simulink model "MotorControlLib"  (R2022b)
settings: Solver=FixedStepDiscrete  StartTime=0.0  StopTime=100  FixedStep=Ts  RelTol=1e-3  EnableMultiTasking=on
values from neighbouring files (symbols this model uses):
  BrkPoints : value not decoded    [MotorControl.sldd]
  CuttOffFreq_c = 4000.0    [MotorControl.sldd]
  d_q_Voltage_Limiter_max = 5.77    [MotorControl.sldd]
  dSoll = 0.0    [MotorControl.sldd]
  EMFobsLdGain = 50000.0    [MotorControl.sldd]
  EMFobsRS = 0.34    [MotorControl.sldd]
  Ki_dAxis = 180.0    [MotorControl.sldd]
  Ki_Iab_EMFobs = 0.0    [MotorControl.sldd]
  Ki_qAxis = 175.0    [MotorControl.sldd]
  Ki_Rpm = 10.0    [MotorControl.sldd]
  Kp_dAxis = 0.146    [MotorControl.sldd]
  Kp_Iab_EMFobs = 1.0    [MotorControl.sldd]
  Kp_qAxis = 0.146    [MotorControl.sldd]
  Kp_Rpm = 0.146    [MotorControl.sldd]
  MaxBckEMFVol_sat_neg = -12.0    [MotorControl.sldd]
  MaxBckEMFVol_sat_pos = 12.0    [MotorControl.sldd]
  Minus_1 = -1.0    [MotorControl.sldd]
  pwmTableData : value not decoded    [MotorControl.sldd]
  TqToIqConst = 1.0    [MotorControl.sldd]
  Ts = 5.0E-5    [MotorControl.sldd]
  TsIntern = 5.0E-5    [MotorControl.sldd]
undefined symbols (not defined in the file or in its folder): DiscIntNeverNeededParam, NumBits1, NumBits2, Slope1, Slope2
libraries: simulink x8, slpidlib x2, simulink_extras x2
(part 1 of 2)
settings Model: DataDictionary=MotorControl.sldd  NumberOfSteps=10  Creator=unix  LastModifiedBy=unix
settings SolverCC: AlgebraicLoopSolver=TrustRegion  AutoInsertRateTranBlk=on
settings OptimizationCC: DefaultParameterBehavior=Inlined  PassReuseOutputArgsAs=Individual arguments  ZeroExternalMemoryAtStartup=off  ZeroInternalMemoryAtStartup=off  EfficientFloat2IntCast=on  OptimizationLevel=level1  OptimizationCustomize=off  EfficientTunableParamExpr=on
settings DebuggingCC: ArrayBoundsChecking=warning  SignalInfNanChecking=warning  SignalRangeChecking=warning  MultiTaskDSMMsg=warning  CheckMatrixSingularityMsg=warning  IntegerOverflowMsg=error  ParameterOverflowMsg=warning  ParameterUnderflowMsg=warning  ParameterPrecisionLossMsg=none  ParameterTunabilityLossMsg=error  UnderSpecifiedDataTypeMsg=warning  UnconnectedInputMsg=warning  UnconnectedOutputMsg=warning  UnconnectedLineMsg=warning  SFMachineParentedDataDiag=warning  IntegerSaturationMsg=error
settings ModelReferenceCC: EnableRefExpFcnMdlSchedulingChecks=on
settings SFSimCC: MATLABDynamicMemAlloc=off
settings RTWCC: Description=Embedded Coder  SystemTargetFile=ert.tlc  GenCodeOnly=on  TemplateMakefile=ert_default_tmf  GenerateReport=on  IncludeHyperlinkInReport=on  LaunchReport=on  GenerateTraceInfo=on  GenerateTraceReport=on  GenerateTraceReportSl=on  GenerateTraceReportSf=on  GenerateTraceReportEml=on  DLArmComputeVersion=19.05
settings CodeAppCC: ForceParamTrailComments=on  IgnoreCustomStorageClasses=off  OperatorAnnotations=on  SimulinkDataObjDesc=on  SFDataObjDesc=on  InsertBlockDesc=on
settings ERTTargetCC: TargetLangStandard=C99 (ISO)  CodeReplacementLibrary=GNU C99 extensions  GenerateSampleERTMain=on  ArrayLayout=Row-major  GenerateASAP2=on  InlinedParameterPlacement=NonHierarchical  ERTCustomFileTemplate=example_file_process.tlc

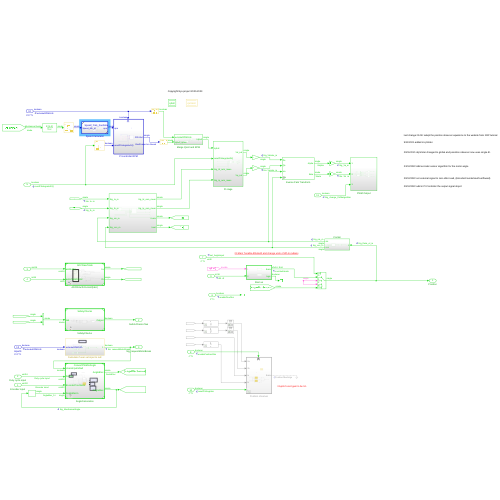
[thumbnail: Simulink's stored preview of the top-level diagram]
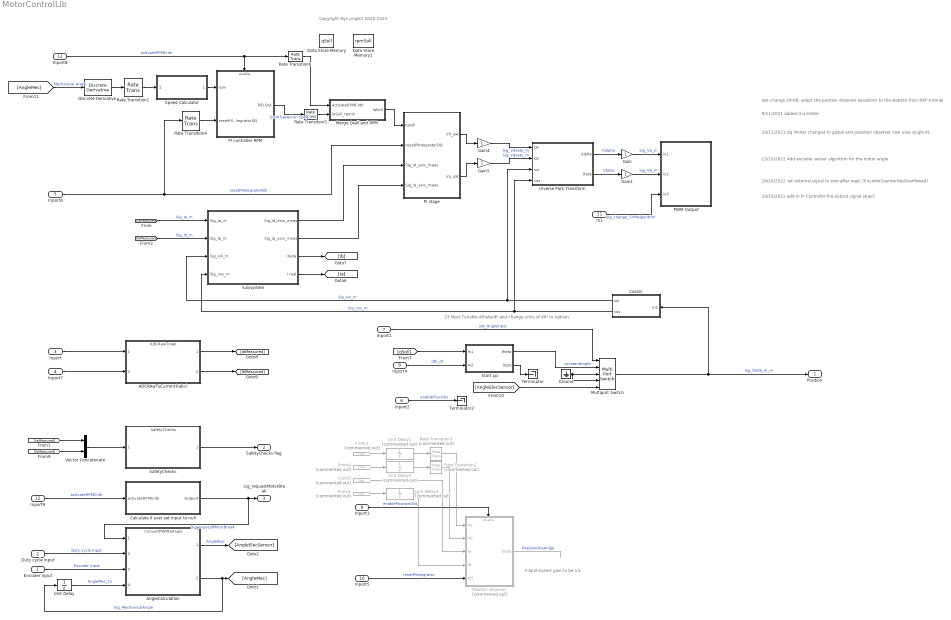
== system MotorControlLib ==
  note: Copyright Nyx project 2020-2023
  note: 29/11/2021 dq limiter changed to global and possition observer now uses single dt.
  note: 9/11/2021 added d-q limiter.
  note: last change 29-08: adapt the position observer equations to the website from NXP tutorial
  note: 3 April-Corect gain to be 1/L
  note: 23 Marz Tunable dtheta/dt and change units of dth to radians
  note: 23/10/2022 Add encoder sensor algorithm for the motor angle
  note: 29/10/2022 set external signal to zero after read, (EncoderCounterHasOverflowed)
  note: 29/10/2022 add in PI Controller the output signal object
  Encoder input : Inport
  Duty cycle input : Inport  Port=2
  Inport : Inport  Port=3
  Inport7 : Inport  Port=4
  Inport6 : Inport  Port=5  OutDataTypeStr=boolean
  Inport2 : Inport  Port=6  OutDataTypeStr=boolean  SampleTime=4*Ts
      settings: AttributesFormatString=%<SampleTime>
  Inport1 : Inport  Port=7  OutDataTypeStr=uint8  SampleTime=4*Ts
      settings: AttributesFormatString=%<SampleTime>
  Inport3 : Inport  Port=8  OutDataTypeStr=boolean  SampleTime=4*Ts
      settings: AttributesFormatString=%<SampleTime>
  Inport4 : Inport  Port=9
  Inport5 : Inport  Port=10  OutDataTypeStr=boolean  SampleTime=4*Ts
      settings: AttributesFormatString=%<SampleTime>
  In1 : Inport  Port=11
  Inport8 : Inport  Port=12  OutDataTypeStr=boolean  SampleTime=200*Ts
      settings: AttributesFormatString=%<SampleTime>
  ADCRAwToCurrent(Iabc) : ModelReference  ModelNameDialog=ADCRawToIab  SimulationMode=Accelerator  ModelReferenceVersion=7.2
  AngleCalculation : ModelReference  ModelNameDialog=ConvertPWMtoAngle.slx  SimulationMode=Accelerator  ModelReferenceVersion=7.35
  Calculate if user set input to null : Subsystem
  CosSin : Subsystem
  Data Store Memory : DataStoreMemory  DataStoreName=qSoll  ReadBeforeWriteMsg=warning  WriteAfterWriteMsg=warning  WriteAfterReadMsg=warning  ShowAdditionalParam=off  StateMustResolveToSignalObject=on
  Data Store Memory1 : DataStoreMemory  DataStoreName=rpmSoll  ReadBeforeWriteMsg=warning  WriteAfterWriteMsg=warning  WriteAfterReadMsg=warning  ShowAdditionalParam=off  StateMustResolveToSignalObject=on
  Discrete Derivative : simulink/Discrete/Discrete Derivative  gainval=1.0  ICPrevScaledInput=0.0  OutMin=[]  OutMax=[]  OutDataType=fixdt(1, 16)  OutScaling=2^-10  DoSatur=off
  From3 : From  Commented=on  GotoTag=Va
  From4 : From  Commented=on  GotoTag=Vb
  From5 : From  Commented=on  GotoTag=Ia
  From6 : From  Commented=on  GotoTag=Ib
  Gain : Gain  OutDataTypeStr=Inherit: Same as input  ParamDataTypeStr=Inherit: Same as input
  Gain1 : Gain  OutDataTypeStr=Inherit: Same as input  ParamDataTypeStr=Inherit: Same as input
  Gain4 : Gain  OutDataTypeStr=Inherit: Inherit via back propagation
  Gain5 : Gain  OutDataTypeStr=Inherit: Inherit via back propagation
  Ground : Ground
  Inport9 : InportShadow  Port=12  OutDataTypeStr=boolean  SampleTime=200*Ts
      settings: AttributesFormatString=%<SampleTime>
  Inverse Park Transform : Subsystem  SystemSampleTime=250*Ts  mask(Inverse Park Transform){AxisAlignment=Q-axis}
      mask prompts: AxisAlignment "Alpha (phase-a) axis alignment:"
      mask help:
      | <p>Compute Inverse Park transformation on rotating reference frame inputs into stationary reference frame outputs.
      | <br><br>
      | The block accepts the following:
      | <ul>
      | <li>d-q axis components in rotating reference frame</li>
      | <li>Sine and cosine values of corresponding angle of transformation</li>
      | </ul>
      | The block outputs &alpha;-&beta; axis components in stationary reference frame.
      | <br><br>
      | D-axis alignment with alpha (phase-a) is popular in motor control theory while Q-axis alignment with alpha (phase-a) is more suitable for power conversion applications.</p>
      mask Help: eval('mcb.internal.helpview(''inverseparktransform'')')
      mask TypeOptions AxisAlignment: D-axis | Q-axis
  Merge Qsoll and RPM : Subsystem
  Multiport Switch : MultiPortSwitch  DataPortOrder=Zero-based contiguous  Inputs=4  zeroidx=on  SaturateOnIntegerOverflow=off  InputSameDT=off
  PI controller RPM : Subsystem  TreatAsAtomicUnit=on  SystemSampleTime=50*Ts
      settings: MinAlgLoopOccurrences=on
  PI stage : Subsystem
  PWM Output : Subsystem
  Position observer : Subsystem  Commented=on
  Rate Transition{1,4..6} (4 alike) : RateTransition  Deterministic=off
  Rate Transition2 : RateTransition  Commented=on
  Rate Transition3 : RateTransition  Commented=on
  SafetyChecks : ModelReference  ModelNameDialog=SafetyChecks.slx  SimulationMode=Accelerator  ModelReferenceVersion=5.3
  Speed Calculator : Subsystem  TreatAsAtomicUnit=on  ReferencedSubsystem=Speed_Calc_FastSlow
      settings: RTWSystemCode=Inline
  Start up : Subsystem  TreatAsAtomicUnit=on  SystemSampleTime=4*Ts
  Subsystem : Subsystem
  Terminator : Terminator
  Terminator2 : Terminator
  Unit Delay : UnitDelay  SampleTime=-1  StateName=AngleMec_1z  HasFrameUpgradeWarning=on  StateMustResolveToSignalObject=on
  Unit Delay1 : UnitDelay  Commented=on  SampleTime=-1  HasFrameUpgradeWarning=on
  Unit Delay2 : UnitDelay  Commented=on  SampleTime=-1  HasFrameUpgradeWarning=on
  Unit Delay3 : UnitDelay  Commented=on  SampleTime=-1  HasFrameUpgradeWarning=on
  Vector Concatenate : Concatenate
  Position : Outport
  SafetyChecks flag : Outport  Port=2
  Sig_requestMotorBreak : Outport  Port=3
  wires:
  Inverse Park Transform/1(Alpha) -> Gain/1  "Valpha"
  Gain4/1 -> Inverse Park Transform/1(Ds)  "Sig_Vdsatu_m"
  Gain5/1 -> Inverse Park Transform/2(Qs)  "Sig_Vqsatu_m"
  Inverse Park Transform/2(Beta) -> Gain1/1  "Vbeta"
  ADCRAwToCurrent(Iabc)/2 -> [IbMeasured]
  Inport/1 -> ADCRAwToCurrent(Iabc)/1
  ADCRAwToCurrent(Iabc)/1 -> [IaMeasured]
  CosSin/1(sin) -> Subsystem/3(Sig_sin_m), Inverse Park Transform/3(sin)  "Sig_sin_m"
  CosSin/2(cos) -> Subsystem/4(Sig_cos_m), Inverse Park Transform/4(cos)  "Sig_cos_m"
  Multiport Switch/1 -> CosSin/1(In1), Position/1  "Sig_theta_el_m"
  Gain/1 -> PWM Output/1(In1)  "Sig_Va_m"
  Gain1/1 -> PWM Output/2(In2)  "Sig_Vb_m"
  [qSoll] -> Start up/1(In1)
  Start up/1(theta) -> Multiport Switch/2  "constantAngle"
  Start up/2(logic) -> Terminator/1
  Inport1/1 -> Multiport Switch/1  "set_AngleInput"
  Inport2/1 -> Terminator2/1  "enableFluxObs"
  Inport3/1 -> Position observer/Enable  "enablePositionObs"
  Position observer/1(theta) -> ?  "PositionObsAnlge"
  Rate Transition2/1 -> Position observer/2(Vb)
  Rate Transition3/1 -> Position observer/1(Va)
  From5/1 -> Position observer/3(Ia)
  Inport4/1 -> Start up/2(In2)  "dth_dt"
  Inport5/1 -> Position observer/5(In5)  "resetPIIntegrator"
  In1/1 -> PWM Output/3(In3)  "Sig_change_SVMalgorithm"
  From4/1 -> Unit Delay2/1
  From3/1 -> Unit Delay1/1
  Vector Concatenate/1 -> SafetyChecks/1
  [IaMeasured] -> Vector Concatenate/1
  [IbMeasured] -> Vector Concatenate/2
  SafetyChecks/1 -> SafetyChecks flag/1
  Inport7/1 -> ADCRAwToCurrent(Iabc)/2
  Duty cycle input/1 -> AngleCalculation/2  "Duty cycle input"
  Unit Delay/1 -> AngleCalculation/4  "AngleMec_1z"
  Encoder input/1 -> AngleCalculation/3  "Encoder input"
  AngleCalculation/2 -> Unit Delay/1, [AngleMec]  "Sig_MechanicalAngle"
  AngleCalculation/1 -> [AngleElecSensor]  "AngleElec"
  [AngleElecSensor] -> Multiport Switch/5
  Unit Delay1/1 -> Rate Transition3/1
  Unit Delay2/1 -> Rate Transition2/1
  From6/1 -> Unit Delay3/1
  Unit Delay3/1 -> Position observer/4(Ib)
  Ground/1 -> Multiport Switch/3, Multiport Switch/4
  Inport6/1 -> PI stage/2(resetPIIntegratorDQ), Rate Transition4/1  "resetPIIntegratorDQ"
  PI stage/1(Vd_sat) -> Gain4/1
  PI stage/2(Vq_sat) -> Gain5/1
  [IaMeasured] -> Subsystem/1(Sig_Ia_m)  "Sig_Ia_m"
  [IbMeasured] -> Subsystem/2(Sig_Ib_m)  "Sig_Ib_m"
  Subsystem/1(Sig_Id_axis_meas) -> PI stage/3(Sig_Id_axis_meas)
  Subsystem/2(Sig_Iq_axis_meas) -> PI stage/4(Sig_Iq_axis_meas)
  Subsystem/3(I beta) -> [Ib]
  Subsystem/4(I real) -> [Ia]
  [AngleMec] -> Discrete Derivative/1  "Mechanical Angle"
  Inport8/1 -> PI controller RPM/Enable, Rate Transition6/1  "activateRPMCntlr"
  PI controller RPM/1(PID Out) -> Rate Transition5/1  "Qsoll based on Speed"
  Merge Qsoll and RPM/1(IqSoll) -> PI stage/1(IqSoll)
  Rate Transition1/1 -> Speed Calculator/1
  Rate Transition4/1 -> PI controller RPM/2(resetPIIntegratorDQ)
  Rate Transition5/1 -> Merge Qsoll and RPM/2(IqSoll_rpmin)
  Discrete Derivative/1 -> Rate Transition1/1
  Calculate if user set input to null/1(Outport) -> Sig_requestMotorBreak/1, AngleCalculation/1  "Sig_requestMotorBreak"
  Inport9/1 -> Calculate if user set input to null/1(activateRPMCntlr)  "activateRPMCntlr"
  Rate Transition6/1 -> Merge Qsoll and RPM/1(activateRPMCntlr)
  Speed Calculator/1 -> PI controller RPM/1(rpm)

== system MotorControlLib/Calculate if user set input to null ==
  note: Set flag if the
      | user Input is Zero.
  activateRPMCntlr : Inport
  AND : Logic  IconShape=distinctive  AllPortsSameDT=off  OutDataTypeStr=boolean
  Compare To Zero : simulink/Logic and Bit Operations/Compare To Zero  relop===  OutDataTypeStr=boolean
  Compare To Zero1 : simulink/Logic and Bit Operations/Compare To Zero  relop===  OutDataTypeStr=boolean
  Data Store Read1 : DataStoreRead  DataStoreName=rpmSoll  IndexOptions=Index vector (dialog)  Indices=1  OutputSizes=1
  Data Store Read2 : DataStoreRead  DataStoreName=qSoll  IndexOptions=Index vector (dialog)  Indices=1  OutputSizes=1
  OR : Logic  Operator=OR  IconShape=distinctive  AllPortsSameDT=off  OutDataTypeStr=boolean
  Outport : Outport
  wires:
  Data Store Read1/1 -> Compare To Zero/1  "qSoll"
  Compare To Zero/1 -> AND/2
  Data Store Read2/1 -> Compare To Zero1/1  "qSoll"
  activateRPMCntlr/1 -> AND/1
  AND/1 -> OR/1
  OR/1 -> Outport/1
  Compare To Zero1/1 -> OR/2

== system MotorControlLib/CosSin ==
  In1 : Inport
  Data Type Conversion1 : DataTypeConversion  SaturateOnIntegerOverflow=off  RndMeth=Floor
  Sine-Cosine Lookup : Subsystem  mask(Sine-Cosine Lookup){AngleInput=Radians, N_points=512}
      mask prompts: AngleInput "Theta units:"; N_points "Number of data points for lookup table:"
      mask help:
      | Implement sine and cosine functions using a lookup table approach for optimized performance on target hardware.
      |
      | The block accepts input angle in different units and outputs corresponding sine and cosine values.
      mask init:
      | % dlgSett = mct.internal.SinCosCb(gcbh);
      | this = get_param(gcbh,'Object');
      | 
      | points = eval(this.N_points);
      | 
      | dlgSett.points = 125*floor(points/125);
      | 
      | dlgSett.Offset = uint16(dlgSett.points/5);
      | 
      | dlgSett.N_points = 4*dlgSett.Offset;
      | N_points = dlgSett.N_points;
      | 
      | theta = linspace(0,2*pi,N_points+1);
      | dlgSett.size = 5*dlgSett.Offset+2;
      | dlgSett.sin_table = zeros(1,dlgSett.size);
      | dlgSett.sin_table(1:N_points+1) = sin(theta);
      | dlgSett.sin_table(N_points+2:dlgSett.size) = dlgSett.sin_table(2:0.25*N_points+2);
      | 
      | dlgSett.N_points = double(dlgSett.N_points);
      | dlgSett.index_gain = dlgSett.N_points;
      | dlgSett.UpperSatLimit = 1;
      | 
      | switch AngleInput
      |     case 1
      |         dlgSett.UpperSatLimit = 1;
      |     case 2
      |         dlgSett.UpperSatLimit = 2*pi;
      |     case 3
      |         dlgSett.UpperSatLimit = 360;
      |     otherwise
      | end
      mask Help: eval('mcb.internal.helpview(''sinecosinelookup'')')
      mask TypeOptions AngleInput: Per-unit | Radians | Degrees
      mask Display: mcb.internal.drawIcons('Sin-Cos',1);
  sin : Outport
  cos : Outport  Port=2
  wires:
  Sine-Cosine Lookup/2(cos) -> cos/1
  In1/1 -> Data Type Conversion1/1
  Sine-Cosine Lookup/1(sin) -> sin/1
  Data Type Conversion1/1 -> Sine-Cosine Lookup/1(Theta)

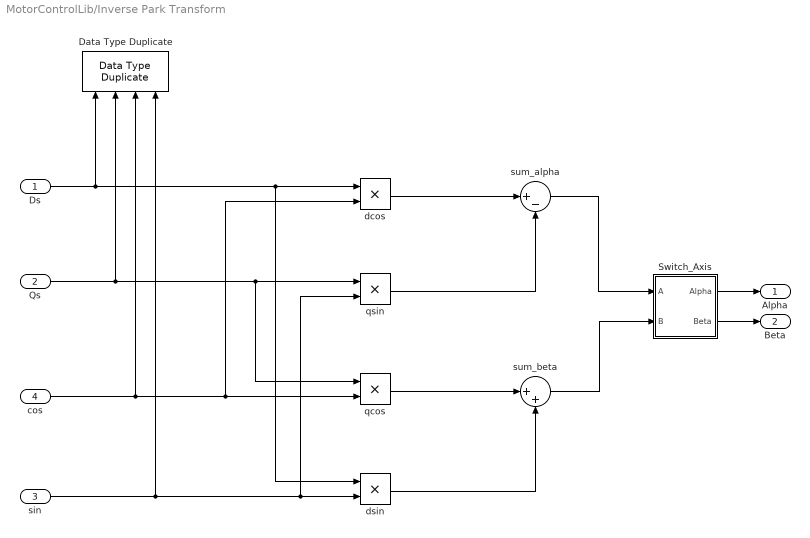
== system MotorControlLib/Inverse Park Transform ==
  Ds : Inport
  Qs : Inport  Port=2
  sin : Inport  Port=3
  cos : Inport  Port=4
  Data Type Duplicate : DataTypeDuplicate  NumInputPorts=4
  Switch_Axis : Subsystem
  dcos : Product  RndMeth=Simplest  OutDataTypeStr=Inherit: Same as first input
  dsin : Product  RndMeth=Simplest  OutDataTypeStr=Inherit: Same as first input
  qcos : Product  RndMeth=Simplest  OutDataTypeStr=Inherit: Same as first input
  qsin : Product  RndMeth=Simplest  OutDataTypeStr=Inherit: Same as first input
  sum_alpha : Sum  Inputs=|+-  RndMeth=Simplest  OutDataTypeStr=Inherit: Same as first input
  sum_beta : Sum  Inputs=|++  RndMeth=Simplest  OutDataTypeStr=Inherit: Same as first input
  Alpha : Outport  VectorParamsAs1DForOutWhenUnconnected=off
  Beta : Outport  Port=2  VectorParamsAs1DForOutWhenUnconnected=off
  wires:
  Switch_Axis/2(Beta) -> Beta/1
  Switch_Axis/1(Alpha) -> Alpha/1
  sum_beta/1 -> Switch_Axis/2(B)
  sum_alpha/1 -> Switch_Axis/1(A)
  sin/1 -> dsin/2, qsin/2, Data Type Duplicate/4
  cos/1 -> qcos/2, dcos/2, Data Type Duplicate/3
  dsin/1 -> sum_beta/2
  Qs/1 -> qsin/1, qcos/1, Data Type Duplicate/2
  dcos/1 -> sum_alpha/1
  qcos/1 -> sum_beta/1
  qsin/1 -> sum_alpha/2
  Ds/1 -> dcos/1, dsin/1, Data Type Duplicate/1

== system MotorControlLib/Merge Qsoll and RPM ==
  activateRPMCntlr : Inport
  IqSoll_rpmin : Inport  Port=2
  Data Store Read : DataStoreRead  DataStoreName=qSoll  IndexOptions=Index vector (dialog)  Indices=1  OutputSizes=1
  Switch : Switch  Criteria=u2 > Threshold  SaturateOnIntegerOverflow=off  InputSameDT=off
  torqueToIq : Subsystem
  IqSoll : Outport
  wires:
  activateRPMCntlr/1 -> Switch/2
  IqSoll_rpmin/1 -> Switch/1
  Data Store Read/1 -> torqueToIq/1(qSoll)  "qSoll"
  Switch/1 -> IqSoll/1  "Sig_Iq_Soll"
  torqueToIq/1(Sig_Iq_Soll) -> Switch/3

== system MotorControlLib/PI controller RPM ==
  rpm : Inport
  resetPIIntegratorDQ : Inport  Port=2
  Enable : EnablePort
  Add : Sum  Inputs=+|-  RndMeth=Simplest
  Constant6 : Constant  Value=Kp_Rpm
  Constant7 : Constant  Value=Ki_Rpm
  Data Store Read1 : DataStoreRead  DataStoreName=rpmSoll  IndexOptions=Index vector (dialog)  Indices=1  OutputSizes=1
  Data Type Conversion3 : DataTypeConversion  OutDataTypeStr=single  SaturateOnIntegerOverflow=off  RndMeth=Floor
  Data Type Conversion4 : DataTypeConversion  OutDataTypeStr=single  SaturateOnIntegerOverflow=off  RndMeth=Floor
  Ground1 : Ground
  PI DAxis : Subsystem  TreatAsAtomicUnit=on  ReferencedSubsystem=PID_custom
  PID Out : Outport
  wires:
  Ground1/1 -> PI DAxis/5
  Data Store Read1/1 -> Add/1  "qSoll"
  Data Type Conversion3/1 -> PI DAxis/2  "Sig_PRPM"
  Data Type Conversion4/1 -> PI DAxis/3  "Sig_IRPM"
  Constant6/1 -> Data Type Conversion3/1
  Constant7/1 -> Data Type Conversion4/1
  Add/1 -> PI DAxis/1
  resetPIIntegratorDQ/1 -> PI DAxis/4
  PI DAxis/1 -> PID Out/1
  rpm/1 -> Add/2  "Sig_Rpm_measurment"

== system MotorControlLib/PI stage ==
  IqSoll : Inport
  resetPIIntegratorDQ : Inport  Port=2
  Sig_Id_axis_meas : Inport  Port=3
  Sig_Iq_axis_meas : Inport  Port=4
  DQ_Limiter : Subsystem  TreatAsAtomicUnit=on  SystemSampleTime=4*Ts  mask(DQ Limiter){Vmax=d_q_Voltage_Limiter_max}
      mask prompts: Vmax "D-Q saturation limit:"
      mask help:
      | Implement saturation on reference dq voltages, with respect to phase voltage peak limit.
      |
      | The block accepts reference values of d and q axis voltages, and outputs corresponding saturated values along with unsaturated peak value to initiate field weakening control.
      |
      | Enter the phase voltage peak limit in the dialog box to initiate saturation.
      settings: RTWFcnNameOpts=Use subsystem name
      mask Help: eval('mcb.internal.helpview(''dqlimiter'')')
  PI_Controller : Subsystem  TreatAsAtomicUnit=on  SystemSampleTime=4*Ts
      settings: RTWFcnNameOpts=Use subsystem name
  Terminator1 : Terminator
  d Soll : Constant  Value=dSoll
  Vd_sat : Outport
  Vq_sat : Outport  Port=2
  wires:
  DQ_Limiter/3(Vmax_unsat) -> Terminator1/1
  d Soll/1 -> PI_Controller/1(dRef)  "dSoll"
  PI_Controller/1(d) -> DQ_Limiter/1(Vd_ref)  "Vdunsat"
  IqSoll/1 -> PI_Controller/2(qRef)
  PI_Controller/2(q) -> DQ_Limiter/2(Vq_ref)  "Vqunsat"
  Sig_Id_axis_meas/1 -> PI_Controller/3(Id_in)
  DQ_Limiter/2(Vq_sat) -> Vq_sat/1
  resetPIIntegratorDQ/1 -> PI_Controller/5(Inport6)
  Sig_Iq_axis_meas/1 -> PI_Controller/4(Iq_in)
  DQ_Limiter/1(Vd_sat) -> Vd_sat/1

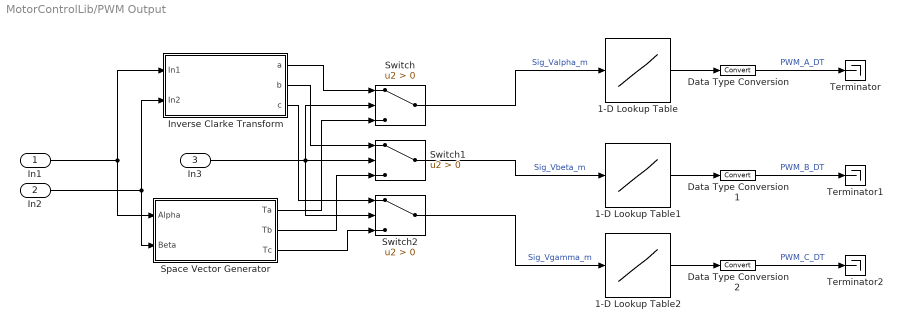
== system MotorControlLib/PWM Output ==
  In1 : Inport
  In2 : Inport  Port=2
  In3 : Inport  Port=3
  1-D Lookup Table : Lookup_n-D  NumberOfTableDimensions=1  BreakpointsForDimension1=BrkPoints  Table=pwmTableData  ExtrapMethod=Clip  InternalRulePriority=Speed  OutDataTypeStr=uint16  RndMeth=Simplest  SaturateOnIntegerOverflow=on
  1-D Lookup Table1 : Lookup_n-D  NumberOfTableDimensions=1  BreakpointsForDimension1=BrkPoints  Table=pwmTableData  ExtrapMethod=Clip  InternalRulePriority=Speed  OutDataTypeStr=uint16  RndMeth=Simplest  SaturateOnIntegerOverflow=on
  1-D Lookup Table2 : Lookup_n-D  NumberOfTableDimensions=1  BreakpointsForDimension1=BrkPoints  Table=pwmTableData  ExtrapMethod=Clip  InternalRulePriority=Speed  OutDataTypeStr=uint16  RndMeth=Simplest  SaturateOnIntegerOverflow=on
  Data Type Conversion : DataTypeConversion  SaturateOnIntegerOverflow=off  RndMeth=Floor
  Data Type Conversion1 : DataTypeConversion  SaturateOnIntegerOverflow=off  RndMeth=Floor
  Data Type Conversion2 : DataTypeConversion  SaturateOnIntegerOverflow=off  RndMeth=Floor
  Inverse Clarke Transform : Subsystem  TreatAsAtomicUnit=on  mask(Inverse Clarke Transform){}
      mask help:
      | <p>Compute Inverse Clarke transformation on balanced 2-phase orthogonal inputs into balanced 3-phase outputs.
      | <br><br>
      | The block accepts &alpha;-&beta; axis components and outputs corresponding 3-phase outputs, where phase-a axis is aligned with &alpha;-axis.</p>
      mask Help: eval('mcb.internal.helpview(''inverseclarketransform'')')
      mask Display: mcb.internal.drawIcons('invClarke',1);
  Space Vector Generator : Subsystem  TreatAsAtomicUnit=on  mask(Space Vector Generator){}
      mask help:
      | <p>Generate space vector modulation signals from stator reference voltages described by  &alpha;-&beta; components.
      | <br><br>
      | The block accepts V<sub>&alpha;</sub> and V<sub>&beta;</sub> voltages and outputs corresponding space vector modulation voltages.</p>
      mask Help: eval('mcb.internal.helpview(''spacevectorgenerator'')')
      mask Display: mcb.internal.drawIcons('SVPWM',1);
  Switch : Switch  Criteria=u2 > Threshold  SaturateOnIntegerOverflow=off  InputSameDT=off
  Switch1 : Switch  Criteria=u2 > Threshold  SaturateOnIntegerOverflow=off  InputSameDT=off
  Switch2 : Switch  Criteria=u2 > Threshold  SaturateOnIntegerOverflow=off  InputSameDT=off
  Terminator : Terminator
  Terminator1 : Terminator
  Terminator2 : Terminator
  wires:
  In2/1 -> Space Vector Generator/2(Beta), Inverse Clarke Transform/2(In2)
  In1/1 -> Space Vector Generator/1(Alpha), Inverse Clarke Transform/1(In1)
  Switch/1 -> 1-D Lookup Table/1  "Sig_Valpha_m"
  1-D Lookup Table/1 -> Data Type Conversion/1
  Switch1/1 -> 1-D Lookup Table1/1  "Sig_Vbeta_m"
  Switch2/1 -> 1-D Lookup Table2/1  "Sig_Vgamma_m"
  1-D Lookup Table2/1 -> Data Type Conversion2/1
  1-D Lookup Table1/1 -> Data Type Conversion1/1
  Data Type Conversion/1 -> Terminator/1  "PWM_A_DT"
  Data Type Conversion1/1 -> Terminator1/1  "PWM_B_DT"
  Data Type Conversion2/1 -> Terminator2/1  "PWM_C_DT"
  Space Vector Generator/1(Ta) -> Switch/3
  Space Vector Generator/2(Tb) -> Switch1/3
  Space Vector Generator/3(Tc) -> Switch2/3
  Inverse Clarke Transform/1(a) -> Switch/1
  Inverse Clarke Transform/2(b) -> Switch1/1
  Inverse Clarke Transform/3(c) -> Switch2/1
  In3/1 -> Switch/2, Switch2/2, Switch1/2

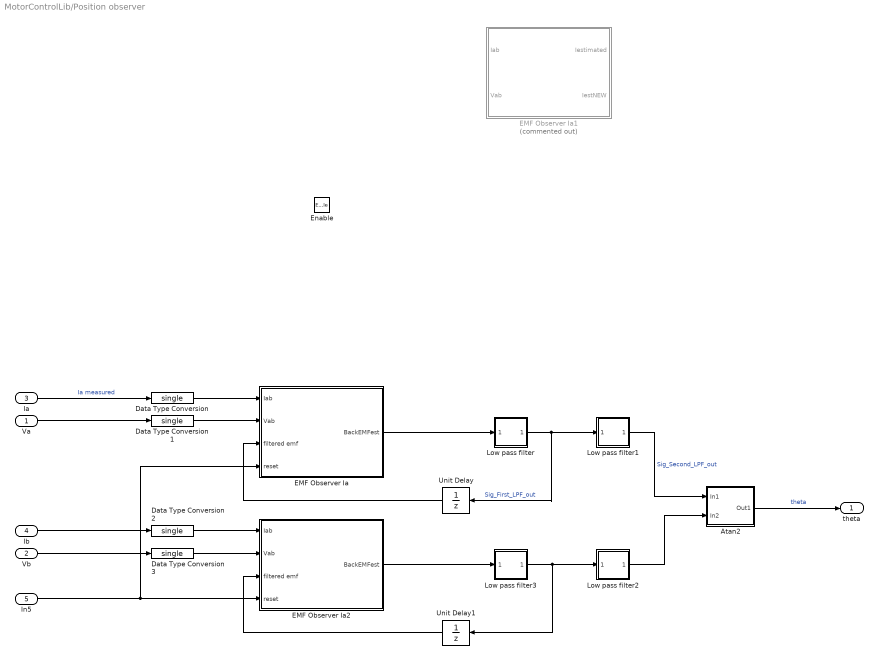
== system MotorControlLib/Position observer ==
  Va : Inport
  Vb : Inport  Port=2
  Ia : Inport  Port=3
  Ib : Inport  Port=4
  In5 : Inport  Port=5
  Enable : EnablePort  StatesWhenEnabling=reset
  Atan2 : Subsystem
  Data Type Conversion{,1..3} (4 alike) : DataTypeConversion  OutDataTypeStr=single  SaturateOnIntegerOverflow=off  RndMeth=Floor
  EMF Observer Ia : Subsystem  mask{Rs=EMFobsRS, Ld=EMFobsLdGain, P=Kp_Iab_EMFobs, I=Ki_Iab_EMFobs}
      mask prompts: Rs "Resistance"; Ld "Inductance"; P "Simulink:masks:ProportionalP_MP"; I "Simulink:masks:IntegralI_MP"
      mask TypeOptions Rs: DC Motor Model/Resistance/Gain
      mask TypeOptions Ld: DC Motor Model/Inductance/Gain
      mask TypeOptions P: PID Controller/P
      mask TypeOptions I: PID Controller/I
      mask DialogControl Container6 Prompt: PI Controller
      mask DialogControl P Prompt: Proportional (P):
      mask DialogControl I Prompt: Integral (I):
  EMF Observer Ia1 : Subsystem  Commented=on  mask{Rs=EMFobsRS, Ld=EMFobsLdGain, P=Kp_Iab_EMFobs, I=Ki_Iab_EMFobs}
      mask prompts: Rs "Resistance"; Ld "Inductance"; P "Simulink:masks:ProportionalP_MP"; I "Simulink:masks:IntegralI_MP"
      mask TypeOptions Rs: DC Motor Model/Resistance/Gain
      mask TypeOptions Ld: DC Motor Model/Inductance/Gain
      mask TypeOptions P: PID Controller/P
      mask TypeOptions I: PID Controller/I
      mask DialogControl Container6 Prompt: PI Controller
      mask DialogControl P Prompt: Proportional (P):
      mask DialogControl I Prompt: Integral (I):
  EMF Observer Ia2 : Subsystem  mask{Rs=EMFobsRS, Ld=EMFobsLdGain, P=Kp_Iab_EMFobs, I=Ki_Iab_EMFobs}
      mask prompts: Rs "Resistance"; Ld "Inductance"; P "Simulink:masks:ProportionalP_MP"; I "Simulink:masks:IntegralI_MP"
      mask TypeOptions Rs: DC Motor Model/Resistance/Gain
      mask TypeOptions Ld: DC Motor Model/Inductance/Gain
      mask TypeOptions P: PID Controller/P
      mask TypeOptions I: PID Controller/I
      mask DialogControl Container6 Prompt: PI Controller
      mask DialogControl P Prompt: Proportional (P):
      mask DialogControl I Prompt: Integral (I):
  Low pass filter : Subsystem  mask{Value=CuttOffFreq_c, Gain=250e-6}
      mask prompts: Value "CuttOff Freq."; Gain "Time interval"
      settings: AttributesFormatString=Integration constant %<Gain>
      mask TypeOptions Value: Constant/Value
      mask TypeOptions Gain: Gain/Gain
  Low pass filter1 : Subsystem  mask{Value=CuttOffFreq_c, Gain=250e-6}
      mask prompts: Value "CuttOff Freq."; Gain "Time interval"
      settings: AttributesFormatString=Integration constant %<Gain>
      mask TypeOptions Value: Constant/Value
      mask TypeOptions Gain: Gain/Gain
  Low pass filter2 : Subsystem  mask{Value=CuttOffFreq_c, Gain=250e-6}
      mask prompts: Value "CuttOff Freq."; Gain "Time interval"
      settings: AttributesFormatString=Integration constant %<Gain>
      mask TypeOptions Value: Constant/Value
      mask TypeOptions Gain: Gain/Gain
  Low pass filter3 : Subsystem  mask{Value=CuttOffFreq_c, Gain=250e-6}
      mask prompts: Value "CuttOff Freq."; Gain "Time interval"
      settings: AttributesFormatString=Integration constant %<Gain>
      mask TypeOptions Value: Constant/Value
      mask TypeOptions Gain: Gain/Gain
  Unit Delay : UnitDelay  SampleTime=-1  HasFrameUpgradeWarning=on
  Unit Delay1 : UnitDelay  SampleTime=-1  HasFrameUpgradeWarning=on
  theta : Outport
  wires:
  Atan2/1(Out1) -> theta/1  "theta"
  Va/1 -> Data Type Conversion1/1
  Ia/1 -> Data Type Conversion/1  "Ia measured"
  Vb/1 -> Data Type Conversion3/1
  Ib/1 -> Data Type Conversion2/1
  EMF Observer Ia/1(BackEMFest) -> Low pass filter/1(In1)
  Low pass filter/1(Output) -> Low pass filter1/1(In1), Unit Delay/1  "Sig_First_LPF_out"
  EMF Observer Ia2/1(BackEMFest) -> Low pass filter3/1(In1)
  Low pass filter3/1(Output) -> Low pass filter2/1(In1), Unit Delay1/1
  Low pass filter1/1(Output) -> Atan2/1(In1)  "Sig_Second_LPF_out"
  Low pass filter2/1(Output) -> Atan2/2(In2)
  Unit Delay/1 -> EMF Observer Ia/3(filtered emf)
  Unit Delay1/1 -> EMF Observer Ia2/3(filtered emf)
  In5/1 -> EMF Observer Ia/4(reset), EMF Observer Ia2/4(reset)
  Data Type Conversion/1 -> EMF Observer Ia/1(Iab)
  Data Type Conversion1/1 -> EMF Observer Ia/2(Vab)
  Data Type Conversion2/1 -> EMF Observer Ia2/1(Iab)
  Data Type Conversion3/1 -> EMF Observer Ia2/2(Vab)

== system MotorControlLib/Start up ==
  In1 : Inport
  In2 : Inport  Port=2
  Logic after motor is stoped : Subsystem
  Simulate start up Theta : Subsystem
  theta : Outport
  logic : Outport  Port=2
  wires:
  In1/1 -> Logic after motor is stoped/1(In1)
  Logic after motor is stoped/1(Out1) -> logic/1
  In2/1 -> Simulate start up Theta/1(In1)
  Simulate start up Theta/1(Out1) -> theta/1

== system MotorControlLib/Subsystem ==
  Sig_Ia_m : Inport
  Sig_Ib_m : Inport  Port=2
  Sig_sin_m : Inport  Port=3
  Sig_cos_m : Inport  Port=4
  Clarke Transform : Subsystem  VariantControl=Variant2  mask(Clarke Transform){}
      mask help:
      | <p>Compute Clarke transformation on balanced 3-phase inputs into balanced 2-phase orthogonal outputs.
      | <br>
      | <br>
      | The block accepts two signals out of three phases, and outputs corresponding &alpha;-&beta; axis components, where phase-a axis is aligned with alpha axis.</p>
      mask Help: eval('mcb.internal.helpview(''clarketransform'')')
      mask Display: mcb.internal.drawIcons('Clarke',1);
  Gain2 : Gain  OutDataTypeStr=Inherit: Same as input  ParamDataTypeStr=Inherit: Same as input
  Gain3 : Gain  OutDataTypeStr=Inherit: Same as input  ParamDataTypeStr=Inherit: Same as input
  Park Transform : Subsystem  SystemSampleTime=250*Ts  mask(Park Transform){AxisAlignment=Q-axis}
      mask prompts: AxisAlignment "Alpha (phase-a) axis alignment:"
      mask help:
      | <p>Compute Park transformation on stationary reference frame inputs into rotating reference frame outputs.
      | <br><br>
      | The block accepts the following:
      | <ul>
      |   <li>&alpha;-&beta; axis components in stationary reference frame</li>
      |   <li>Sine and cosine values of corresponding angle of transformation</li>
      | </ul>
      | The block outputs direct and quadrature axis components in rotating reference frame.
      | <br><br>
      | D-axis alignment with alpha (phase-a) is popular in motor control theory while Q-axis alignment with alpha (phase-a) is more suitable for power conversion applications.</p>
      mask Help: eval('mcb.internal.helpview(''parktransform'')')
      mask TypeOptions AxisAlignment: D-axis | Q-axis
  Sig_Id_axis_meas : Outport
  Sig_Iq_axis_meas : Outport  Port=2
  I beta : Outport  Port=3
  I real : Outport  Port=4
  wires:
  Clarke Transform/2(Beta) -> I beta/1, Park Transform/2(Beta)  "Sig_Ibeta_m"
  Park Transform/2(Qs) -> Gain3/1  "Iq"
  Clarke Transform/1(Alpha) -> I real/1, Park Transform/1(Alpha)  "I real"
  Sig_cos_m/1 -> Park Transform/4(cos)
  Sig_Ia_m/1 -> Clarke Transform/1(a)
  Sig_Ib_m/1 -> Clarke Transform/2(b)
  Park Transform/1(Ds) -> Gain2/1  "Id"
  Sig_sin_m/1 -> Park Transform/3(sine)
  Gain3/1 -> Sig_Iq_axis_meas/1  "Sig_Iq_axis_meas"
  Gain2/1 -> Sig_Id_axis_meas/1  "Sig_Id_axis_meas"

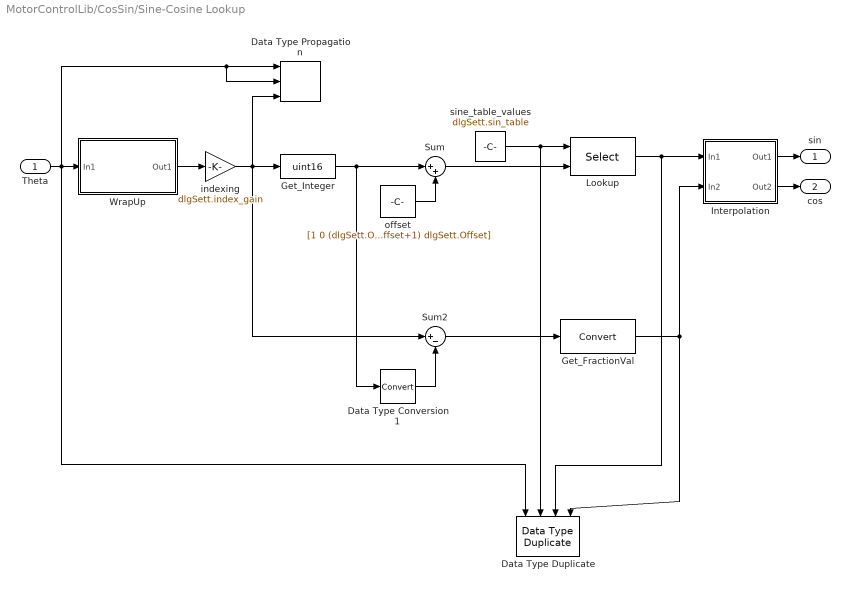
== system MotorControlLib/CosSin/Sine-Cosine Lookup ==
  Theta : Inport
  Data Type Duplicate : DataTypeDuplicate  NumInputPorts=4
  Data Type Propagation : simulink/Signal Attributes/Data Type Propagation  PropDataType=fixdt(1, 16)  IfRefDouble=double  IfRefSingle=single  IsSigned=IsSigned1 or IsSigned2  NumBitsBase=max([NumBits1 NumBits2])  NumBitsMult=1  NumBitsAdd=0  NumBitsAllowFinal=1:128  PropScalingMode=Obtain via best precision  PropScaling=2^-10  ValuesUsedBestPrec=[0 dlgSett.index_gain]  SlopeBase=min([Slope1 Slope2])  SlopeMult=1  SlopeAdd=0  BiasBase=Bias1  BiasMult=1  BiasAdd=0
  Data Type Conversion1 : DataTypeConversion  RndMeth=Simplest  SaturateOnIntegerOverflow=off
  Get_FractionVal : DataTypeConversion  RndMeth=Simplest  SaturateOnIntegerOverflow=off
  Get_Integer : DataTypeConversion  OutDataTypeStr=uint16  RndMeth=Simplest  SaturateOnIntegerOverflow=off
  Interpolation : Subsystem
  Lookup : Selector  IndexMode=Zero-based  InputPortWidth=dlgSett.size  IndexOptions=Index vector (port)  Indices=[1 3]  OutputSizes=1
  Sum : Sum  Inputs=|++  AccumDataTypeStr=uint32  OutDataTypeStr=uint32  RndMeth=Simplest
  Sum2 : Sum  Inputs=|+-  RndMeth=Simplest  OutDataTypeStr=Inherit: Same as first input
  WrapUp : Subsystem
  indexing : Gain  Gain=dlgSett.index_gain  OutDataTypeStr=Inherit: Inherit via back propagation  RndMeth=Simplest
  offset : Constant  Value=[1 0 (dlgSett.Offset+1) dlgSett.Offset]  OutDataTypeStr=int16  SampleTime=-1
  sine_table_values : Constant  Value=dlgSett.sin_table  OutDataTypeStr=Inherit: Inherit via back propagation  SampleTime=-1
  sin : Outport  VectorParamsAs1DForOutWhenUnconnected=off
  cos : Outport  Port=2  VectorParamsAs1DForOutWhenUnconnected=off
  wires:
  Interpolation/2(Out2) -> cos/1
  Interpolation/1(Out1) -> sin/1
  Sum/1 -> Lookup/2
  indexing/1 -> Sum2/1, Data Type Propagation/3, Get_Integer/1
  Data Type Conversion1/1 -> Sum2/2
  Get_Integer/1 -> Sum/1, Data Type Conversion1/1
  offset/1 -> Sum/2
  sine_table_values/1 -> Lookup/1, Data Type Duplicate/2
  Lookup/1 -> Interpolation/1(In1), Data Type Duplicate/3
  Sum2/1 -> Get_FractionVal/1
  Get_FractionVal/1 -> Data Type Duplicate/4, Interpolation/2(In2)
  Theta/1 -> Data Type Duplicate/1, WrapUp/1(In1), Data Type Propagation/2, Data Type Propagation/1
  WrapUp/1(Out1) -> indexing/1

== system MotorControlLib/Inverse Park Transform/Switch_Axis ==
  A : Inport
  B : Inport  Port=2
  D_axis_aligned : Mux  Inputs=2
  Demux : Demux  Outputs=2
  Offset : Constant  Value=0  OutDataTypeStr=uint16  SampleTime=-1
  Q_axis_aligned : Mux  Inputs=2
  Switch : Switch  Criteria=u2 > Threshold  Threshold=1  RndMeth=Simplest  ZeroCross=off  SaturateOnIntegerOverflow=off  InputSameDT=off
  Unary_Minus : UnaryMinus
  Alpha : Outport  VectorParamsAs1DForOutWhenUnconnected=off
  Beta : Outport  Port=2  VectorParamsAs1DForOutWhenUnconnected=off
  wires:
  A/1 -> D_axis_aligned/1, Unary_Minus/1
  Unary_Minus/1 -> Q_axis_aligned/2
  Demux/2 -> Beta/1
  Switch/1 -> Demux/1
  B/1 -> D_axis_aligned/2, Q_axis_aligned/1
  Demux/1 -> Alpha/1
  Offset/1 -> Switch/2
  Q_axis_aligned/1 -> Switch/1
  D_axis_aligned/1 -> Switch/3

== system MotorControlLib/Merge Qsoll and RPM/torqueToIq ==
  qSoll : Inport
  Tq--> iqRef : Gain  Gain=TqToIqConst  ParamDataTypeStr=Inherit: Inherit from 'Gain'  OutDataTypeStr=single
  Sig_Iq_Soll : Outport
  wires:
  Tq--> iqRef/1 -> Sig_Iq_Soll/1
  qSoll/1 -> Tq--> iqRef/1

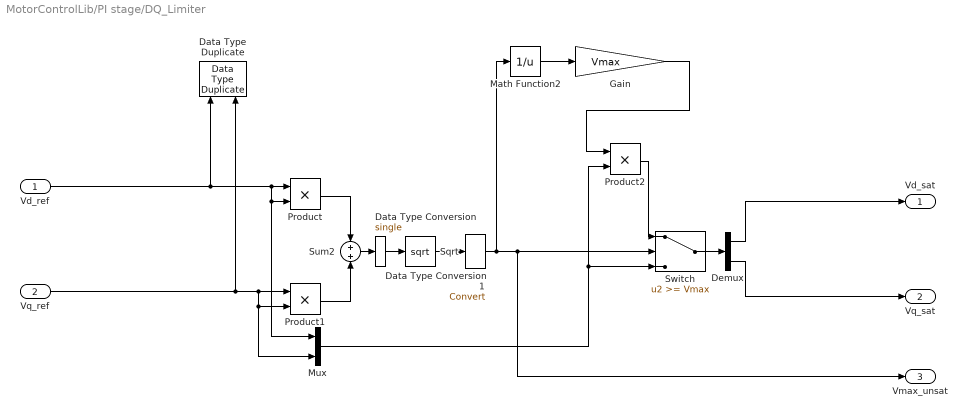
== system MotorControlLib/PI stage/DQ_Limiter ==
  Vd_ref : Inport
  Vq_ref : Inport  Port=2
  Data Type Duplicate : DataTypeDuplicate
  Data Type Conversion : DataTypeConversion  OutDataTypeStr=single  SaturateOnIntegerOverflow=off  RndMeth=Floor
  Data Type Conversion1 : DataTypeConversion  SaturateOnIntegerOverflow=off  RndMeth=Floor
  Demux : Demux  Outputs=2
  Gain : Gain  Gain=Vmax  OutDataTypeStr=Inherit: Same as input
  Math Function2 : Math  Operator=reciprocal  SignedPower=on  RndMeth=Simplest  SaturateOnIntegerOverflow=off
  Mux : Mux  Inputs=2
  Product : Product  RndMeth=Simplest  OutDataTypeStr=Inherit: Same as first input
  Product1 : Product  RndMeth=Simplest  OutDataTypeStr=Inherit: Same as first input
  Product2 : Product  OutDataTypeStr=Inherit: Same as first input
  Sqrt : Sqrt  IntermediateResultsDataTypeStr=Inherit: Inherit from input
  Sum2 : Sum  OutDataTypeStr=Inherit: Same as first input
  Switch : Switch  Threshold=Vmax  ZeroCross=off  SaturateOnIntegerOverflow=off  InputSameDT=off
  Vd_sat : Outport  VectorParamsAs1DForOutWhenUnconnected=off
  Vq_sat : Outport  Port=2  VectorParamsAs1DForOutWhenUnconnected=off
  Vmax_unsat : Outport  Port=3  VectorParamsAs1DForOutWhenUnconnected=off
  wires:
  Vd_ref/1 -> Data Type Duplicate/1, Product/1, Product/2, Mux/1
  Demux/1 -> Vd_sat/1
  Product1/1 -> Sum2/2
  Product/1 -> Sum2/1
  Sum2/1 -> Data Type Conversion/1
  Math Function2/1 -> Gain/1
  Mux/1 -> Product2/2, Switch/3
  Product2/1 -> Switch/1
  Switch/1 -> Demux/1
  Demux/2 -> Vq_sat/1
  Sqrt/1 -> Data Type Conversion1/1
  Gain/1 -> Product2/1
  Vq_ref/1 -> Data Type Duplicate/2, Product1/1, Product1/2, Mux/2
  Data Type Conversion1/1 -> Vmax_unsat/1, Switch/2, Math Function2/1
  Data Type Conversion/1 -> Sqrt/1

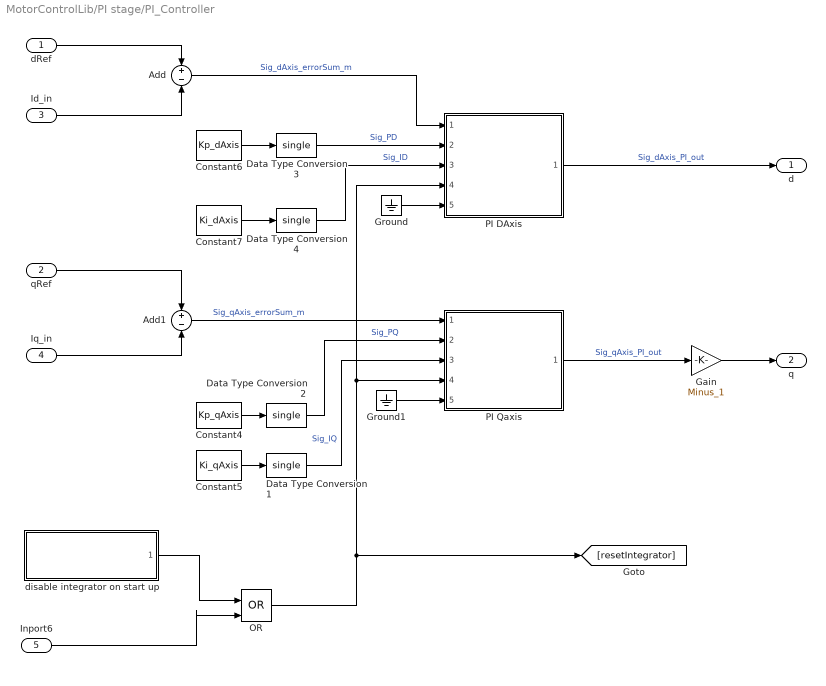
== system MotorControlLib/PI stage/PI_Controller ==
  dRef : Inport
  qRef : Inport  Port=2
  Id_in : Inport  Port=3
  Iq_in : Inport  Port=4
  Inport6 : Inport  Port=5
  Add : Sum  Inputs=+|-  RndMeth=Simplest
  Add1 : Sum  Inputs=+|-  RndMeth=Simplest
  Constant4 : Constant  Value=Kp_qAxis
  Constant5 : Constant  Value=Ki_qAxis
  Constant6 : Constant  Value=Kp_dAxis
  Constant7 : Constant  Value=Ki_dAxis
  Data Type Conversion{1..4} (4 alike) : DataTypeConversion  OutDataTypeStr=single  SaturateOnIntegerOverflow=off  RndMeth=Floor
  Gain : Gain  Gain=Minus_1
  Ground : Ground
  Ground1 : Ground
  OR : Logic  Operator=OR  IconShape=distinctive  AllPortsSameDT=off  OutDataTypeStr=boolean
  PI DAxis : Subsystem  TreatAsAtomicUnit=on  ReferencedSubsystem=PID_custom
  PI Qaxis : Subsystem  TreatAsAtomicUnit=on  ReferencedSubsystem=PID_custom
  disable integrator on start up : Subsystem  ReferencedSubsystem=disable_integrator_on_start_up
  d : Outport
  q : Outport  Port=2
  wires:
  dRef/1 -> Add/1
  qRef/1 -> Add1/1
  Iq_in/1 -> Add1/2
  PI Qaxis/1 -> Gain/1  "Sig_qAxis_PI_out"
  Id_in/1 -> Add/2
  Add1/1 -> PI Qaxis/1  "Sig_qAxis_errorSum_m"
  Constant5/1 -> Data Type Conversion1/1
  Constant4/1 -> Data Type Conversion2/1
  disable integrator on start up/1 -> OR/1
  Inport6/1 -> OR/2
  Data Type Conversion1/1 -> PI Qaxis/3  "Sig_IQ"
  Data Type Conversion2/1 -> PI Qaxis/2  "Sig_PQ"
  Add/1 -> PI DAxis/1  "Sig_dAxis_errorSum_m"
  Constant6/1 -> Data Type Conversion3/1
  Constant7/1 -> Data Type Conversion4/1
  PI DAxis/1 -> d/1  "Sig_dAxis_PI_out"
  OR/1 -> [resetIntegrator], PI DAxis/4, PI Qaxis/4
  Data Type Conversion3/1 -> PI DAxis/2  "Sig_PD"
  Data Type Conversion4/1 -> PI DAxis/3  "Sig_ID"
  Ground/1 -> PI DAxis/5
  Ground1/1 -> PI Qaxis/5
  Gain/1 -> q/1

== system MotorControlLib/PWM Output/Inverse Clarke Transform ==
  In1 : Inport
  In2 : Inport  Port=2
  Data Type Duplicate : DataTypeDuplicate
  add_b : Sum  Inputs=-+  RndMeth=Simplest  OutDataTypeStr=Inherit: Same as first input
  add_c : Sum  Inputs=--  RndMeth=Simplest  OutDataTypeStr=Inherit: Same as first input
  one_by_two : Gain  Gain=1/2  RndMeth=Simplest  OutDataTypeStr=Inherit: Same as input
  sqrt3_by_two : Gain  Gain=sqrt(3)/2  RndMeth=Simplest  OutDataTypeStr=Inherit: Same as input
  a : Outport  VectorParamsAs1DForOutWhenUnconnected=off
  b : Outport  Port=2  VectorParamsAs1DForOutWhenUnconnected=off
  c : Outport  Port=3  VectorParamsAs1DForOutWhenUnconnected=off
  wires:
  add_c/1 -> c/1
  sqrt3_by_two/1 -> add_c/2, add_b/2
  In1/1 -> one_by_two/1, Data Type Duplicate/1, a/1
  one_by_two/1 -> add_b/1, add_c/1
  In2/1 -> sqrt3_by_two/1, Data Type Duplicate/2
  add_b/1 -> b/1

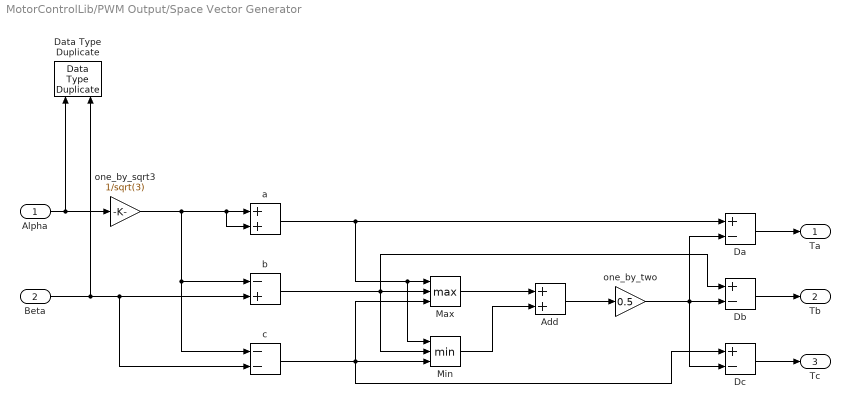
== system MotorControlLib/PWM Output/Space Vector Generator ==
  Alpha : Inport
  Beta : Inport  Port=2
  Add : Sum  RndMeth=Simplest  OutDataTypeStr=Inherit: Same as first input
  Da : Sum  Inputs=+-  RndMeth=Simplest  OutDataTypeStr=Inherit: Same as first input
  Data Type Duplicate : DataTypeDuplicate
  Db : Sum  Inputs=+-  RndMeth=Simplest  OutDataTypeStr=Inherit: Same as first input
  Dc : Sum  Inputs=+-  RndMeth=Simplest  OutDataTypeStr=Inherit: Same as first input
  Max : MinMax  Function=max  Inputs=3  RndMeth=Simplest
  Min : MinMax  Inputs=3  RndMeth=Simplest
  a : Sum  RndMeth=Simplest  OutDataTypeStr=Inherit: Same as first input
  b : Sum  Inputs=-+  RndMeth=Simplest  OutDataTypeStr=Inherit: Same as first input
  c : Sum  Inputs=--  RndMeth=Simplest  OutDataTypeStr=Inherit: Same as first input
  one_by_sqrt3 : Gain  Gain=1/sqrt(3)  RndMeth=Simplest  OutDataTypeStr=Inherit: Same as input  ParamDataTypeStr=Inherit: Same as input
  one_by_two : Gain  Gain=0.5  RndMeth=Simplest  OutDataTypeStr=Inherit: Same as input  ParamDataTypeStr=Inherit: Same as input
  Ta : Outport  VectorParamsAs1DForOutWhenUnconnected=off
  Tb : Outport  Port=2  VectorParamsAs1DForOutWhenUnconnected=off
  Tc : Outport  Port=3  VectorParamsAs1DForOutWhenUnconnected=off
  wires:
  Db/1 -> Tb/1
  Dc/1 -> Tc/1
  Da/1 -> Ta/1
  a/1 -> Max/1, Min/1, Da/1
  Max/1 -> Add/1
  one_by_two/1 -> Da/2, Db/2, Dc/2
  Add/1 -> one_by_two/1
  Min/1 -> Add/2
  Alpha/1 -> Data Type Duplicate/1, one_by_sqrt3/1
  one_by_sqrt3/1 -> a/1, a/2, b/1, c/1
  Beta/1 -> c/2, b/2, Data Type Duplicate/2
  b/1 -> Max/2, Min/2, Db/1
  c/1 -> Min/3, Dc/1, Max/3

== system MotorControlLib/Position observer/Atan2 ==
  In1 : Inport
  In2 : Inport  Port=2
  Atan2 : Trigonometry  Operator=atan2  ApproximationMethod=CORDIC  NumberOfIterations=6
  Data Type Conversion5 : DataTypeConversion  SaturateOnIntegerOverflow=off  RndMeth=Floor
  Data Type Conversion6 : DataTypeConversion  OutDataTypeStr=single  SaturateOnIntegerOverflow=off  RndMeth=Floor
  Data Type Conversion7 : DataTypeConversion  OutDataTypeStr=single  SaturateOnIntegerOverflow=off  RndMeth=Floor
  Out1 : Outport
  wires:
  Atan2/1 -> Data Type Conversion5/1
  In1/1 -> Data Type Conversion6/1
  Data Type Conversion6/1 -> Atan2/1
  Data Type Conversion7/1 -> Atan2/2
  In2/1 -> Data Type Conversion7/1
  Data Type Conversion5/1 -> Out1/1

== system MotorControlLib/Position observer/EMF Observer Ia ==
  Iab : Inport
  Vab : Inport  Port=2
  filtered emf : Inport  Port=3
  reset : Inport  Port=4
  Add6 : Sum  Inputs=-+  InputSameDT=on
  DC Motor Model : Subsystem  TreatAsAtomicUnit=on  SystemSampleTime=Ts
  PI Controller : Subsystem
  Rate Transition{,1..3} (4 alike) : RateTransition  Integrity=off
  Unit Delay : UnitDelay  SampleTime=-1  HasFrameUpgradeWarning=on
  BackEMFest : Outport
  wires:
  Iab/1 -> Add6/1
  DC Motor Model/1(i_integrated_en8) -> Rate Transition/1
  Vab/1 -> Rate Transition1/1
  Rate Transition/1 -> Add6/2  "Iest"
  Rate Transition1/1 -> DC Motor Model/2(In2)
  Rate Transition2/1 -> DC Motor Model/1(Sig_Emfobs_PI_out)
  PI Controller/1(Sig_Emfobs_PI_out) -> Unit Delay/1, BackEMFest/1  "BackEMF est"
  Add6/1 -> PI Controller/1(Sig_Emfobs_errorSum_m)  "Sig_Emfobs_errorSum_m"
  filtered emf/1 -> Rate Transition3/1
  Rate Transition3/1 -> DC Motor Model/3(In3)
  Unit Delay/1 -> Rate Transition2/1
  reset/1 -> PI Controller/2(reset)

== system MotorControlLib/Position observer/EMF Observer Ia1 ==
  Iab : Inport
  Vab : Inport  Port=2
  DC Motor Model : Subsystem
  PI Controller : Subsystem
  Rate Transition : RateTransition
  Rate Transition1 : RateTransition
  Rate Transition2 : RateTransition
  Unit Delay : UnitDelay  SampleTime=-1  HasFrameUpgradeWarning=on
  Iestimated : Outport
  IestNEW : Outport  Port=2
  wires:
  DC Motor Model/1(Out1) -> Rate Transition/1
  Vab/1 -> Rate Transition1/1
  Rate Transition/1 -> PI Controller/2(In2), IestNEW/1
  Rate Transition1/1 -> DC Motor Model/2(In2)
  Rate Transition2/1 -> DC Motor Model/1(In1)
  PI Controller/1(Out1) -> Iestimated/1, Unit Delay/1
  Iab/1 -> PI Controller/1(In1)
  Unit Delay/1 -> Rate Transition2/1

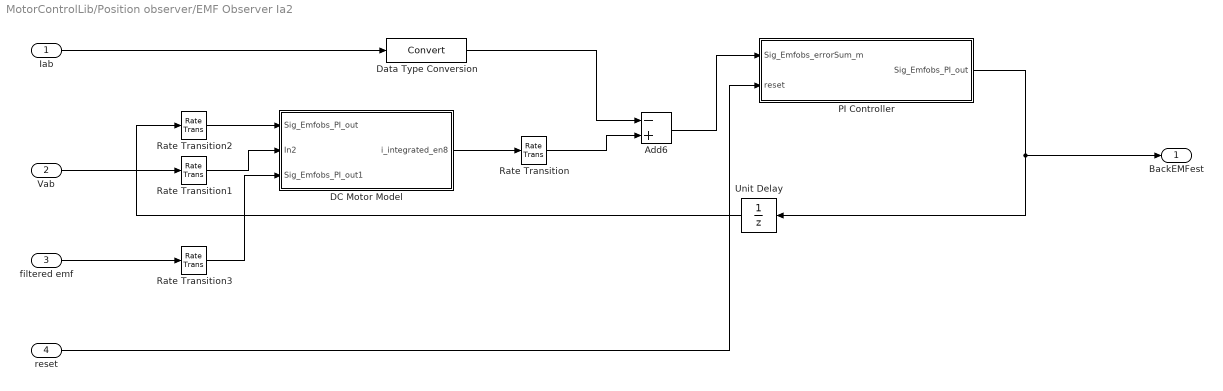
== system MotorControlLib/Position observer/EMF Observer Ia2 ==
  Iab : Inport
  Vab : Inport  Port=2
  filtered emf : Inport  Port=3
  reset : Inport  Port=4
  Add6 : Sum  Inputs=-+  InputSameDT=on
  DC Motor Model : Subsystem  TreatAsAtomicUnit=on  SystemSampleTime=Ts
  Data Type Conversion : DataTypeConversion  SaturateOnIntegerOverflow=off  RndMeth=Floor
  PI Controller : Subsystem  TreatAsAtomicUnit=on
  Rate Transition{,1..3} (4 alike) : RateTransition  Integrity=off
  Unit Delay : UnitDelay  SampleTime=-1  HasFrameUpgradeWarning=on
  BackEMFest : Outport
  wires:
  PI Controller/1(Sig_Emfobs_PI_out) -> Unit Delay/1, BackEMFest/1
  Add6/1 -> PI Controller/1(Sig_Emfobs_errorSum_m)
  Rate Transition2/1 -> DC Motor Model/1(Sig_Emfobs_PI_out)
  Rate Transition1/1 -> DC Motor Model/2(In2)
  Rate Transition/1 -> Add6/2
  Vab/1 -> Rate Transition1/1
  DC Motor Model/1(i_integrated_en8) -> Rate Transition/1
  Iab/1 -> Data Type Conversion/1
  Data Type Conversion/1 -> Add6/1
  filtered emf/1 -> Rate Transition3/1
  Rate Transition3/1 -> DC Motor Model/3(Sig_Emfobs_PI_out1)
  Unit Delay/1 -> Rate Transition2/1
  reset/1 -> PI Controller/2(reset)

== system MotorControlLib/Position observer/Low pass filter ==
  note: Integrator
  note: d/dt(i)
  In1 : Inport
  Add2 : Sum  Inputs=+-
  Constant : Constant  Value=Value  OutDataTypeStr=uint16
  Delay : Delay  DelayLength=1  InitialCondition=0
  Gain : Gain  Gain=Gain  ParamDataTypeStr=fixdt(1,16,2^-16,0)  OutDataTypeStr=fixdt(1,16,2^-14,0)  SaturateOnIntegerOverflow=on
  Product1 : Product  OutDataTypeStr=fixdt(1,16,2^-6,0)
  Sum : Sum  Inputs=|++  OutDataTypeStr=Inherit: Same as first input
  Unit Delay : UnitDelay  SampleTime=-1  HasFrameUpgradeWarning=on
  Output : Outport
  wires:
  Constant/1 -> Product1/2
  In1/1 -> Add2/1
  Add2/1 -> Gain/1
  Product1/1 -> Output/1, Unit Delay/1
  Gain/1 -> Sum/1
  Delay/1 -> Sum/2
  Sum/1 -> Delay/1, Product1/1
  Unit Delay/1 -> Add2/2

== system MotorControlLib/Position observer/Low pass filter1 ==
  note: d/dt(i)
  note: Integrator
  In1 : Inport
  Add2 : Sum  Inputs=+-
  Constant : Constant  Value=Value  OutDataTypeStr=uint16
  Delay : Delay  DelayLength=1  InitialCondition=0
  Gain : Gain  Gain=Gain  ParamDataTypeStr=fixdt(1,16,2^-16,0)  OutDataTypeStr=fixdt(1,16,2^-14,0)  SaturateOnIntegerOverflow=on
  Product1 : Product  OutDataTypeStr=fixdt(1,16,2^-6,0)
  Sum : Sum  Inputs=|++  OutDataTypeStr=Inherit: Same as first input
  Unit Delay : UnitDelay  SampleTime=-1  HasFrameUpgradeWarning=on
  Output : Outport
  wires:
  Unit Delay/1 -> Add2/2
  Sum/1 -> Product1/1, Delay/1
  Delay/1 -> Sum/2
  Gain/1 -> Sum/1
  Product1/1 -> Unit Delay/1, Output/1
  Add2/1 -> Gain/1
  In1/1 -> Add2/1
  Constant/1 -> Product1/2

== system MotorControlLib/Position observer/Low pass filter2 ==
  note: Integrator
  note: d/dt(i)
  In1 : Inport
  Add2 : Sum  Inputs=+-
  Constant : Constant  Value=Value  OutDataTypeStr=uint16
  Delay : Delay  DelayLength=1  InitialCondition=0
  Gain : Gain  Gain=Gain  ParamDataTypeStr=fixdt(1,16,2^-16,0)  OutDataTypeStr=fixdt(1,16,2^-14,0)  SaturateOnIntegerOverflow=on
  Product1 : Product  OutDataTypeStr=fixdt(1,16,2^-6,0)
  Sum : Sum  Inputs=|++  OutDataTypeStr=Inherit: Same as first input
  Unit Delay : UnitDelay  SampleTime=-1  HasFrameUpgradeWarning=on
  Output : Outport
  wires:
  Constant/1 -> Product1/2
  In1/1 -> Add2/1
  Add2/1 -> Gain/1
  Product1/1 -> Output/1, Unit Delay/1
  Gain/1 -> Sum/1
  Delay/1 -> Sum/2
  Sum/1 -> Delay/1, Product1/1
  Unit Delay/1 -> Add2/2

== system MotorControlLib/Position observer/Low pass filter3 ==
  note: d/dt(i)
  note: Integrator
  In1 : Inport
  Add2 : Sum  Inputs=+-
  Constant : Constant  Value=Value  OutDataTypeStr=uint16
  Delay : Delay  DelayLength=1  InitialCondition=0
  Gain : Gain  Gain=Gain  ParamDataTypeStr=fixdt(1,16,2^-16,0)  OutDataTypeStr=fixdt(1,16,2^-14,0)  SaturateOnIntegerOverflow=on
  Product1 : Product  OutDataTypeStr=fixdt(1,16,2^-6,0)
  Sum : Sum  Inputs=|++  OutDataTypeStr=Inherit: Same as first input
  Unit Delay : UnitDelay  SampleTime=-1  HasFrameUpgradeWarning=on
  Output : Outport
  wires:
  Unit Delay/1 -> Add2/2
  Sum/1 -> Product1/1, Delay/1
  Delay/1 -> Sum/2
  Gain/1 -> Sum/1
  Product1/1 -> Unit Delay/1, Output/1
  Add2/1 -> Gain/1
  In1/1 -> Add2/1
  Constant/1 -> Product1/2

== system MotorControlLib/Start up/Logic after motor is stoped ==
  In1 : Inport
  Compare To Zero : simulink/Logic and Bit Operations/Compare To Zero  relop===  OutDataTypeStr=boolean
  Detect Decrease : simulink/Logic and Bit Operations/Detect Decrease  vinit=0  OutDataTypeStr=boolean
  Enabled Subsystem : Subsystem  TreatAsAtomicUnit=on
  Enabled Subsystem1 : Subsystem  TreatAsAtomicUnit=on
  S-R Flip-Flop : simulink_extras/Flip Flops/S-R Flip-Flop  initial_condition=0
  S-R Flip-Flop1 : simulink_extras/Flip Flops/S-R Flip-Flop  initial_condition=0
  Terminator : Terminator
  Terminator1 : Terminator
  Unit Delay : UnitDelay  SampleTime=-1  HasFrameUpgradeWarning=on
  Unit Delay1 : UnitDelay  SampleTime=-1  HasFrameUpgradeWarning=on
  Out1 : Outport
  wires:
  Enabled Subsystem/1(Out1) -> S-R Flip-Flop1/1
  In1/1 -> Enabled Subsystem/1(In1), Compare To Zero/1
  S-R Flip-Flop/2 -> Terminator/1
  Enabled Subsystem1/1(Output) -> Out1/1, Unit Delay1/1
  S-R Flip-Flop/1 -> Enabled Subsystem/Enable
  S-R Flip-Flop1/1 -> Enabled Subsystem1/Enable, Unit Delay/1
  Unit Delay/1 -> S-R Flip-Flop/2
  Compare To Zero/1 -> S-R Flip-Flop/1
  S-R Flip-Flop1/2 -> Terminator1/1
  Unit Delay1/1 -> Detect Decrease/1
  Detect Decrease/1 -> S-R Flip-Flop1/2

== system MotorControlLib/Start up/Simulate start up Theta ==
  note: Overflow danger
  In1 : Inport
  Abs : Abs  SaturateOnIntegerOverflow=off
  Constant : Constant  Value=2*pi  OutDataTypeStr=fixdt(1,16,2^-8,0)
  Discrete-Time Integrator : DiscreteIntegrator  ExternalReset=rising  SampleTime=-1  OutDataTypeStr=fixdt(1,16,2^-8,0)  ICPrevOutput=DiscIntNeverNeededParam  ICPrevScaledInput=DiscIntNeverNeededParam
  Relational Operator : RelationalOperator  OutDataTypeStr=boolean  RndMeth=Simplest  InputSameDT=off
  Unit Delay : UnitDelay  SampleTime=-1  HasFrameUpgradeWarning=on
  Out1 : Outport
  wires:
  Constant/1 -> Relational Operator/2
  Relational Operator/1 -> Unit Delay/1
  Unit Delay/1 -> Discrete-Time Integrator/2
  In1/1 -> Discrete-Time Integrator/1
  Discrete-Time Integrator/1 -> Out1/1, Abs/1
  Abs/1 -> Relational Operator/1

== system MotorControlLib/Subsystem/Clarke Transform ==
  a : Inport
  b : Inport  Port=2
  Data Type Duplicate : DataTypeDuplicate
  a_plus_2b : Sum  Inputs=+++  RndMeth=Simplest  OutDataTypeStr=Inherit: Same as first input
  one_by_sqrt3 : Gain  Gain=1/sqrt(3)  RndMeth=Simplest  OutDataTypeStr=Inherit: Same as input
  Alpha : Outport  VectorParamsAs1DForOutWhenUnconnected=off
  Beta : Outport  Port=2  VectorParamsAs1DForOutWhenUnconnected=off
  wires:
  a/1 -> a_plus_2b/1, Alpha/1, Data Type Duplicate/1
  one_by_sqrt3/1 -> Beta/1
  a_plus_2b/1 -> one_by_sqrt3/1
  b/1 -> a_plus_2b/2, a_plus_2b/3, Data Type Duplicate/2
